simulink model "Problem2"  (R2020b)
settings: Solver=VariableStepAuto  StartTime=0.0  StopTime=10.0  RelTol=1e-3
model workspace (MAT data in the model file):
  Fn = [0  0; 1  0.8; 2  1.6; 3  1.6; 4  1.6; 5  1.6; 6  0.8; 7  0; 8  0; 9  0; 10  0]
  Ie = 1
  Iv = 5
  R = 1
  Tin = [1  2; 2  2; 3  2; 4  2; 5  2; 6  0; 7  0; 8  0; 9  0; 10  0]
  be = 2
  bv = 1
  f1 = [1; 6; 11; 16; 21; 26; 31; 36; 41; 46; 51]
  muk = 1
  mus = 1.5
settings Model: OrderedModelArguments=off  Creator=HP  LastModifiedBy=Admin

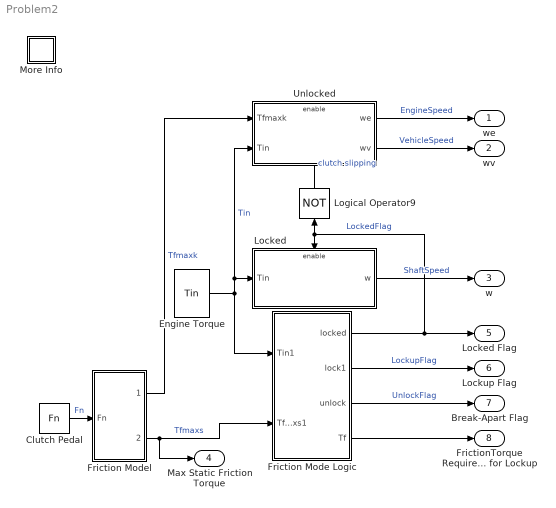
== system Problem2 ==
  Clutch Pedal : FromWorkspace  VariableName=Fn  ZeroCross=off
  Engine Torque : FromWorkspace  VariableName=Tin  ZeroCross=off
  Friction Model : Subsystem
  Friction Mode Logic : Subsystem
      mask Display: plot([-3 1 1 3 -1 -1],[-1 -1 1 1 1 -1],-4,-5,4,5)
  Locked : Subsystem  TreatAsAtomicUnit=on
      mask Display: plot(-1,-6,6,12,[0 3],[3 3],[3 1 1 3], [1 1 5 5],[2 4 4 2],[4 4 2 2],[4 5],[3 3])
  Logical Operator9 : Logic  Operator=NOT  Inputs=1  IconShape=distinctive  OutDataTypeStr=boolean
  More Info : Subsystem
      settings: OpenFcn=showExample('simulink_automotive/BuildingAClutchLockUpModelExample')
      mask Display: disp('?')
  Unlocked : Subsystem  TreatAsAtomicUnit=on
      mask Display: plot(-1,-2,6,8,[0 3],[3 3],[3 1 1 3], [1 1 5 5],[2 4 4 2],[4 4 2 2],[4 5],[3 3])
  we : Outport  InitialOutput=0  VectorParamsAs1DForOutWhenUnconnected=off
  wv : Outport  Port=2  InitialOutput=0  VectorParamsAs1DForOutWhenUnconnected=off
  w : Outport  Port=3  InitialOutput=0  VectorParamsAs1DForOutWhenUnconnected=off
  Max Static Friction Torque : Outport  Port=4  InitialOutput=0  VectorParamsAs1DForOutWhenUnconnected=off
  Locked Flag : Outport  Port=5  InitialOutput=0  VectorParamsAs1DForOutWhenUnconnected=off
  Lockup Flag : Outport  Port=6  InitialOutput=0  VectorParamsAs1DForOutWhenUnconnected=off
  Break-Apart Flag : Outport  Port=7  InitialOutput=0  VectorParamsAs1DForOutWhenUnconnected=off
  FrictionTorque Required for Lockup : Outport  Port=8  InitialOutput=0  VectorParamsAs1DForOutWhenUnconnected=off
  wires:
  Friction Model/2(Tfmaxs) -> Friction Mode Logic/2(Tfmaxs1), Max Static Friction Torque/1  "Tfmaxs"
  Clutch Pedal/1 -> Friction Model/1(Fn)  "Fn"
  Logical Operator9/1 -> Unlocked/Enable  "clutch slipping"
  Engine Torque/1 -> Friction Mode Logic/1(Tin1), Unlocked/2(Tin), Locked/1(Tin)  "Tin"
  Unlocked/2(wv) -> wv/1  "VehicleSpeed"
  Friction Model/1(Tfmaxk) -> Unlocked/1(Tfmaxk)  "Tfmaxk"
  Locked/1(w) -> w/1  "ShaftSpeed"
  Unlocked/1(we) -> we/1  "EngineSpeed"
  Friction Mode Logic/2(lock1) -> Lockup Flag/1  "LockupFlag"
  Friction Mode Logic/1(locked) -> Locked Flag/1, Logical Operator9/1, Locked/Enable  "LockedFlag"
  Friction Mode Logic/4(Tf) -> FrictionTorque Required for Lockup/1
  Friction Mode Logic/3(unlock) -> Break-Apart Flag/1  "UnlockFlag"

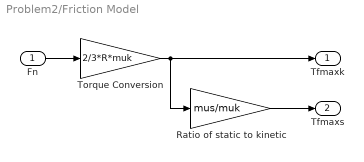
== system Problem2/Friction Model ==
  Fn : Inport
  Ratio of static to kinetic : Gain  Gain=mus/muk  SaturateOnIntegerOverflow=on  OutDataTypeStr=Inherit: Same as input  ParamDataTypeStr=Inherit: Same as input
  Torque Conversion : Gain  Gain=2/3*R*muk  SaturateOnIntegerOverflow=on  OutDataTypeStr=Inherit: Same as input  ParamDataTypeStr=Inherit: Same as input
  Tfmaxk : Outport  InitialOutput=0  VectorParamsAs1DForOutWhenUnconnected=off
  Tfmaxs : Outport  Port=2  InitialOutput=0  VectorParamsAs1DForOutWhenUnconnected=off
  wires:
  Torque Conversion/1 -> Tfmaxk/1, Ratio of static to kinetic/1
  Fn/1 -> Torque Conversion/1
  Ratio of static to kinetic/1 -> Tfmaxs/1

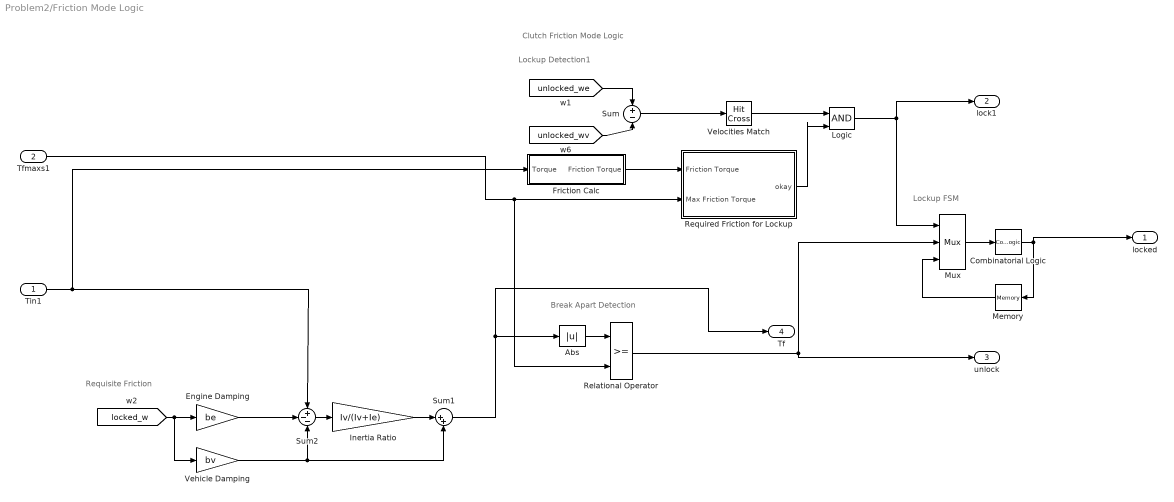
== system Problem2/Friction Mode Logic ==
  note: Lockup FSM
  note: Break Apart
      | Detection
  note: Requisite Friction
  note: Lockup
      | Detection1
  note: Clutch Friction Mode Logic
  Tin1 : Inport
  Tfmaxs1 : Inport  Port=2
  Abs : Abs  SaturateOnIntegerOverflow=on
  Combinatorial Logic : CombinatorialLogic  TruthTable=[0;1;0;0;1;1;1;0]
  Engine Damping : Gain  Gain=be  SaturateOnIntegerOverflow=on  OutDataTypeStr=Inherit: Same as input  ParamDataTypeStr=Inherit: Same as input
  Friction Calc : Subsystem
  Inertia Ratio : Gain  Gain=Iv/(Iv+Ie)  SaturateOnIntegerOverflow=on  OutDataTypeStr=Inherit: Same as input  ParamDataTypeStr=Inherit: Same as input
  Logic : Logic  IconShape=distinctive  OutDataTypeStr=boolean
  Memory : Memory
  Mux : Mux  Inputs=3
  Relational Operator : RelationalOperator  OutDataTypeStr=boolean  RndMeth=Nearest  InputSameDT=on
  Required Friction for Lockup : Subsystem
  Sum : Sum  Inputs=+-  InputSameDT=on  SaturateOnIntegerOverflow=on  OutDataTypeStr=Inherit: Same as first input
  Sum1 : Sum  Inputs=|++  InputSameDT=on  SaturateOnIntegerOverflow=on  OutDataTypeStr=Inherit: Same as first input
  Sum2 : Sum  Inputs=+--  InputSameDT=on  SaturateOnIntegerOverflow=on  OutDataTypeStr=Inherit: Same as first input
  Vehicle Damping : Gain  Gain=bv  SaturateOnIntegerOverflow=on  OutDataTypeStr=Inherit: Same as input  ParamDataTypeStr=Inherit: Same as input
  Velocities Match : HitCross
  locked : Outport  InitialOutput=0  VectorParamsAs1DForOutWhenUnconnected=off
  lock1 : Outport  Port=2  InitialOutput=0  VectorParamsAs1DForOutWhenUnconnected=off
  unlock : Outport  Port=3  InitialOutput=0  VectorParamsAs1DForOutWhenUnconnected=off
  Tf : Outport  Port=4  InitialOutput=0  VectorParamsAs1DForOutWhenUnconnected=off
  wires:
  Combinatorial Logic/1 -> locked/1, Memory/1
  Sum/1 -> Velocities Match/1
  [unlocked_wv] -> Sum/2
  [unlocked_we] -> Sum/1
  Required Friction for Lockup/1(okay) -> Logic/2
  Velocities Match/1 -> Logic/1
  Friction Calc/1(Friction Torque) -> Required Friction for Lockup/1(Friction Torque)
  Inertia Ratio/1 -> Sum1/1
  Tin1/1 -> Sum2/1, Friction Calc/1(Torque)
  Sum2/1 -> Inertia Ratio/1
  Vehicle Damping/1 -> Sum2/3, Sum1/2
  Engine Damping/1 -> Sum2/2
  [locked_w] -> Vehicle Damping/1, Engine Damping/1
  Tfmaxs1/1 -> Relational Operator/2, Required Friction for Lockup/2(Max Friction Torque)
  Abs/1 -> Relational Operator/1
  Sum1/1 -> Tf/1, Abs/1
  Mux/1 -> Combinatorial Logic/1
  Logic/1 -> Mux/1, lock1/1
  Relational Operator/1 -> Mux/2, unlock/1
  Memory/1 -> Mux/3

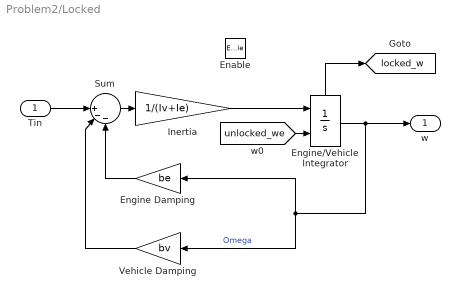
== system Problem2/Locked ==
  Tin : Inport
  Enable : EnablePort  StatesWhenEnabling=reset
  Engine Damping : Gain  Gain=be  SaturateOnIntegerOverflow=on  OutDataTypeStr=Inherit: Same as input  ParamDataTypeStr=Inherit: Same as input
  Engine/Vehicle Integrator : Integrator  InitialConditionSource=external  ShowStatePort=on
  Inertia : Gain  Gain=1/(Iv+Ie)  SaturateOnIntegerOverflow=on  OutDataTypeStr=Inherit: Same as input  ParamDataTypeStr=Inherit: Same as input
  Sum : Sum  Inputs=||+--  InputSameDT=on  SaturateOnIntegerOverflow=on  OutDataTypeStr=Inherit: Same as first input
  Vehicle Damping : Gain  Gain=bv  SaturateOnIntegerOverflow=on  OutDataTypeStr=Inherit: Same as input  ParamDataTypeStr=Inherit: Same as input
  w : Outport  InitialOutput=0  VectorParamsAs1DForOutWhenUnconnected=off
  tag scope: locked_w=global
  wires:
  [unlocked_we] -> Engine/Vehicle Integrator/2
  Engine/Vehicle Integrator/State -> [locked_w]
  Sum/1 -> Inertia/1
  Tin/1 -> Sum/1
  Engine/Vehicle Integrator/1 -> w/1, Engine Damping/1, Vehicle Damping/1  "Omega"
  Engine Damping/1 -> Sum/3
  Inertia/1 -> Engine/Vehicle Integrator/1
  Vehicle Damping/1 -> Sum/2

== system Problem2/More Info ==

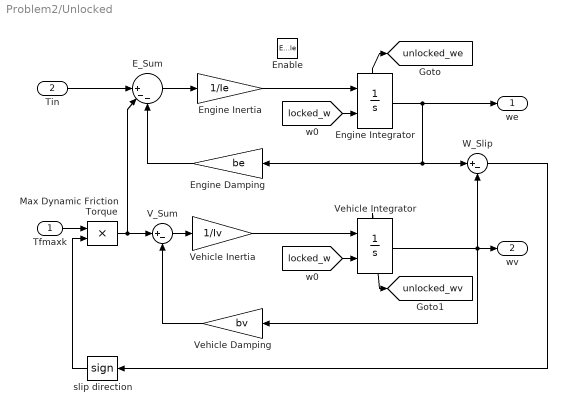
== system Problem2/Unlocked ==
  Tfmaxk : Inport
  Tin : Inport  Port=2
  Enable : EnablePort  StatesWhenEnabling=reset
  E_Sum : Sum  Inputs=||+--  InputSameDT=on  SaturateOnIntegerOverflow=on  OutDataTypeStr=Inherit: Same as first input
  Engine Damping : Gain  Gain=be  SaturateOnIntegerOverflow=on  OutDataTypeStr=Inherit: Same as input  ParamDataTypeStr=Inherit: Same as input
  Engine Inertia : Gain  Gain=1/Ie  SaturateOnIntegerOverflow=on  OutDataTypeStr=Inherit: Same as input  ParamDataTypeStr=Inherit: Same as input
  Engine Integrator : Integrator  InitialConditionSource=external  ShowStatePort=on
  Max Dynamic Friction Torque : Product  InputSameDT=on  RndMeth=Zero  SaturateOnIntegerOverflow=on  OutDataTypeStr=Inherit: Same as first input
  V_Sum : Sum  Inputs=|+-  InputSameDT=on  SaturateOnIntegerOverflow=on  OutDataTypeStr=Inherit: Same as first input
  Vehicle Damping : Gain  Gain=bv  SaturateOnIntegerOverflow=on  OutDataTypeStr=Inherit: Same as input  ParamDataTypeStr=Inherit: Same as input
  Vehicle Inertia : Gain  Gain=1/Iv  SaturateOnIntegerOverflow=on  OutDataTypeStr=Inherit: Same as input  ParamDataTypeStr=Inherit: Same as input
  Vehicle Integrator : Integrator  InitialConditionSource=external  ShowStatePort=on
  W_Slip : Sum  Inputs=|+-  InputSameDT=on  SaturateOnIntegerOverflow=on  OutDataTypeStr=Inherit: Same as first input
  slip direction : Signum
  we : Outport  InitialOutput=0  VectorParamsAs1DForOutWhenUnconnected=off
  wv : Outport  Port=2  InitialOutput=0  VectorParamsAs1DForOutWhenUnconnected=off
  tag scope: unlocked_we=global, unlocked_wv=global
  wires:
  V_Sum/1 -> Vehicle Inertia/1
  Vehicle Damping/1 -> V_Sum/2
  Max Dynamic Friction Torque/1 -> V_Sum/1, E_Sum/2
  Tfmaxk/1 -> Max Dynamic Friction Torque/1
  slip direction/1 -> Max Dynamic Friction Torque/2
  W_Slip/1 -> slip direction/1
  Engine Integrator/State -> [unlocked_we]
  Engine Inertia/1 -> Engine Integrator/1
  E_Sum/1 -> Engine Inertia/1
  Engine Damping/1 -> E_Sum/3
  Engine Integrator/1 -> we/1, Engine Damping/1, W_Slip/1
  [locked_w] -> Engine Integrator/2
  Tin/1 -> E_Sum/1
  Vehicle Integrator/State -> [unlocked_wv]
  [locked_w] -> Vehicle Integrator/2
  Vehicle Inertia/1 -> Vehicle Integrator/1
  Vehicle Integrator/1 -> Vehicle Damping/1, wv/1, W_Slip/2

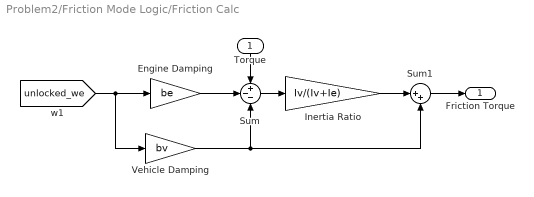
== system Problem2/Friction Mode Logic/Friction Calc ==
  Torque : Inport
  Engine Damping : Gain  Gain=be  SaturateOnIntegerOverflow=on  OutDataTypeStr=Inherit: Same as input  ParamDataTypeStr=Inherit: Same as input
  Inertia Ratio : Gain  Gain=Iv/(Iv+Ie)  SaturateOnIntegerOverflow=on  OutDataTypeStr=Inherit: Same as input  ParamDataTypeStr=Inherit: Same as input
  Sum : Sum  Inputs=+--  InputSameDT=on  SaturateOnIntegerOverflow=on  OutDataTypeStr=Inherit: Same as first input
  Sum1 : Sum  Inputs=|++  InputSameDT=on  SaturateOnIntegerOverflow=on  OutDataTypeStr=Inherit: Same as first input
  Vehicle Damping : Gain  Gain=bv  SaturateOnIntegerOverflow=on  OutDataTypeStr=Inherit: Same as input  ParamDataTypeStr=Inherit: Same as input
  Friction Torque : Outport  InitialOutput=0  VectorParamsAs1DForOutWhenUnconnected=off
  wires:
  [unlocked_we] -> Engine Damping/1, Vehicle Damping/1
  Vehicle Damping/1 -> Sum1/2, Sum/3
  Engine Damping/1 -> Sum/2
  Sum/1 -> Inertia Ratio/1
  Torque/1 -> Sum/1
  Inertia Ratio/1 -> Sum1/1
  Sum1/1 -> Friction Torque/1

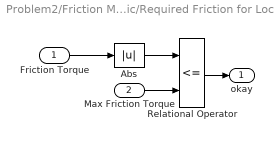
== system Problem2/Friction Mode Logic/Required Friction for Lockup ==
  Friction Torque : Inport
  Max Friction Torque : Inport  Port=2
  Abs : Abs  SaturateOnIntegerOverflow=on
  Relational Operator : RelationalOperator  Operator=<=  OutDataTypeStr=boolean  RndMeth=Nearest  InputSameDT=on
  okay : Outport  InitialOutput=0  VectorParamsAs1DForOutWhenUnconnected=off
  wires:
  Friction Torque/1 -> Abs/1
  Relational Operator/1 -> okay/1
  Abs/1 -> Relational Operator/1
  Max Friction Torque/1 -> Relational Operator/2
